simulink subsystem "Handlebar_Interface_Board"  (R2023b)
settings: Solver=VariableStepAuto  StartTime=0.0  StopTime=10.0  RelTol=1e-3
settings Model: Creator=heyka  LastModifiedBy=heyka
settings DebuggingCC: UnconnectedInputMsg=warning  UnconnectedOutputMsg=warning  UnconnectedLineMsg=warning
settings ModelReferenceCC: EnableRefExpFcnMdlSchedulingChecks=on
settings RTWCC: DLArmComputeVersion=19.05

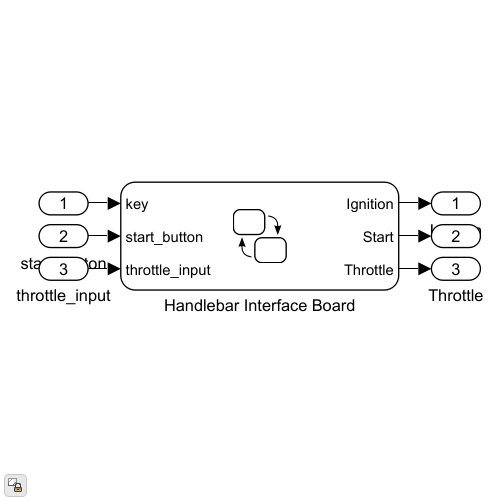
[thumbnail: Simulink's stored preview of the top-level diagram]
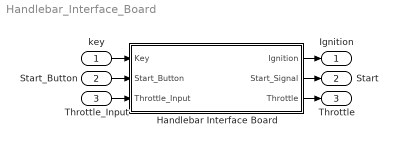
== system Handlebar_Interface_Board ==
  key : Inport
  Start_Button : Inport  Port=2
  Throttle_Input : Inport  Port=3
  Handlebar Interface Board : Stateflow chart  TreatAsAtomicUnit=on
  Ignition : Outport
  Start : Outport  Port=2
  Throttle : Outport  Port=3
  wires:
  Handlebar Interface Board/2(Start_Signal) -> Start/1
  Handlebar Interface Board/3(Throttle) -> Throttle/1
  Start_Button/1 -> Handlebar Interface Board/2(Start_Button)
  Handlebar Interface Board/1(Ignition) -> Ignition/1
  key/1 -> Handlebar Interface Board/1(Key)
  Throttle_Input/1 -> Handlebar Interface Board/3(Throttle_Input)

== stateflow chart Handlebar_Interface_Board/Handlebar Interface Board ==
  state Ignition_OFF
    during:
    Ignition = 0
    Throttle = 0
    Start_Signal = 0
  state Ignition_ON
    during:
    Ignition = 1
    Start_Signal = 0
  state Bike_Start
    during:
    Ignition = 1
    Start_Signal = 1
    Throttle = Throttle_Input
  (default) -> Ignition_OFF
  Ignition_OFF -> Ignition_ON : [Key == 1]
  Ignition_ON -> Ignition_OFF [order 2] : [Key == 0]
  Bike_Start -> Ignition_ON [order 1] : [Start_Button == 0]
  Ignition_ON -> Bike_Start [order 1] : [Start_Button== 1]
  Bike_Start -> Ignition_OFF [order 2] : [Key == 0]
  data: Ignition output =0; Start_Signal output =0; Key input; Start_Button input; Throttle output =0; Throttle_Input input
